simulink library "Plane_Movement_stand_still"  (R2024a)
settings: Solver=VariableStepAuto  StartTime=0.0  StopTime=10.0  RelTol=1e-3
undefined symbols (not defined in the file): Lower_limbs, Upper_limbs
libraries: functionAngles x1
settings Model: Creator=renre  LastModifiedBy=renre

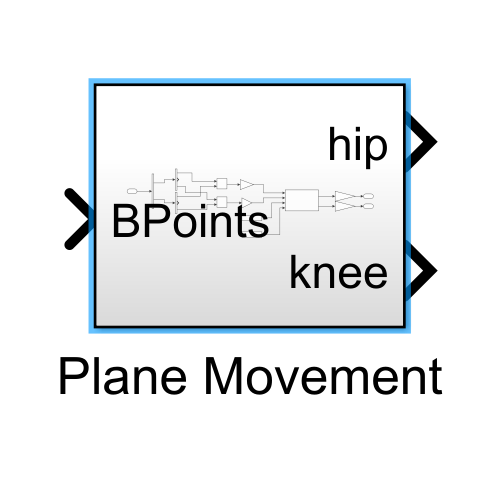
[thumbnail: Simulink's stored preview of the top-level diagram]
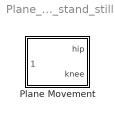
== system Plane_Movement_stand_still ==
  Plane Movement : Subsystem

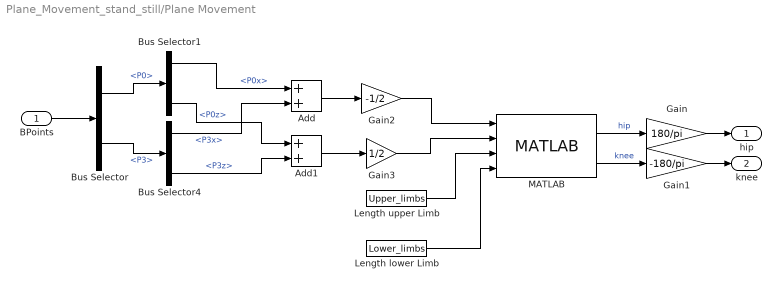
== system Plane_Movement_stand_still/Plane Movement ==
  BPoints : Inport
  Add : Sum
  Add1 : Sum
  Bus Selector : BusSelector  OutputSignals=P0,P3
  Bus Selector1 : BusSelector  OutputSignals=P0x,P0y,P0z
  Bus Selector4 : BusSelector  OutputSignals=P3x,P3y,P3z
  Gain : Gain  Gain=180/pi
  Gain1 : Gain  Gain=-180/pi
  Gain2 : Gain  Gain=-1/2
  Gain3 : Gain  Gain=1/2
  Length lower Limb : Constant  Value=Lower_limbs
  Length upper Limb : Constant  Value=Upper_limbs
  MATLAB : functionAngles/MATLAB  SystemSampleTime=-1  VariantActivationTime=update diagram  AllowFlexibleInterface=on  Latency=0  AutoFrameSizeCalculation=off
  hip : Outport
  knee : Outport  Port=2
  wires:
  Bus Selector1/3 -> Add1/1  "<P0z>"
  Bus Selector1/1 -> Add/1  "<P0x>"
  Bus Selector/2 -> Bus Selector4/1  "<P3>"
  Bus Selector/1 -> Bus Selector1/1  "<P0>"
  MATLAB/2 -> Gain1/1  "knee"
  MATLAB/1 -> Gain/1  "hip"
  Length upper Limb/1 -> MATLAB/3
  Length lower Limb/1 -> MATLAB/4
  Gain1/1 -> knee/1
  Gain/1 -> hip/1
  Bus Selector4/1 -> Add/2  "<P3x>"
  Gain3/1 -> MATLAB/2
  Bus Selector4/3 -> Add1/2  "<P3z>"
  Add/1 -> Gain2/1
  Add1/1 -> Gain3/1
  Gain2/1 -> MATLAB/1
  BPoints/1 -> Bus Selector/1
